simulink model "Ejercicio2_CustomFuzzyBlock"  (R2025a)
settings: Solver=ode8  StartTime=0.0  StopTime=10.0  FixedStep=0.01  RelTol=1e-3
libraries: fuzblock x1
settings Model: Creator=zokra  LastModifiedBy=440G5

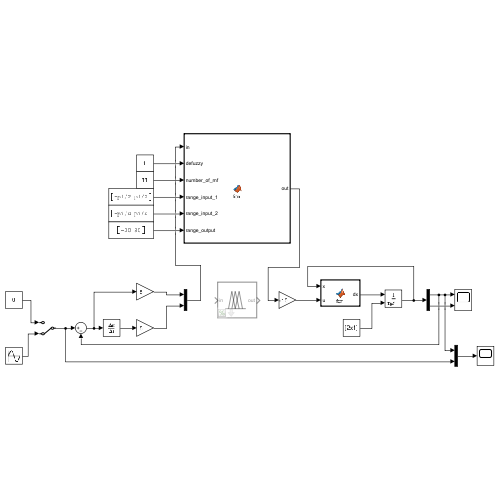
[thumbnail: Simulink's stored preview of the top-level diagram]
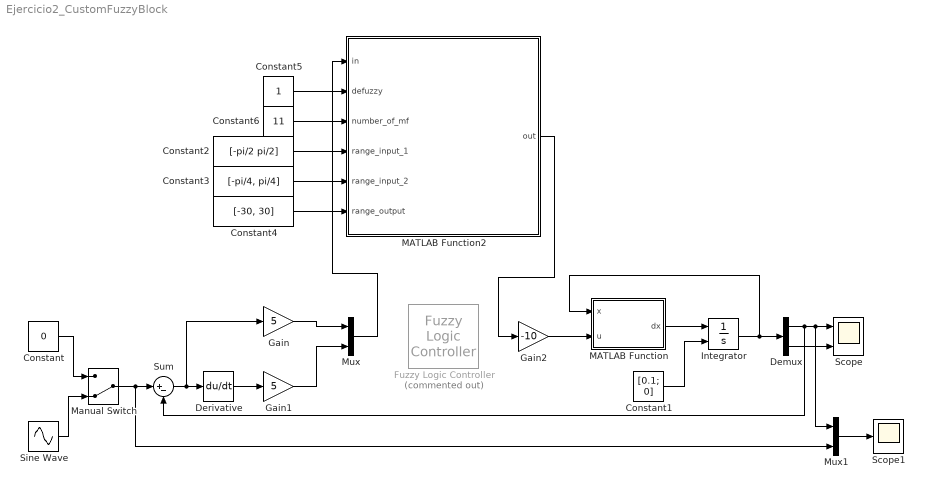
== system Ejercicio2_CustomFuzzyBlock ==
  Constant : Constant  Value=0
  Constant1 : Constant  Value=[0.1; 0]
  Constant2 : Constant  Value=[-pi/2 pi/2]
  Constant3 : Constant  Value=[-pi/4, pi/4]
  Constant4 : Constant  Value=[-30, 30]
  Constant5 : Constant
  Constant6 : Constant  Value=11
  Demux : Demux  Outputs=2
  Derivative : Derivative
  Fuzzy Logic Controller : fuzblock/Fuzzy Logic  Controller  Commented=on  FIS='25_rules_4.fis'  OutputSampleNumber=101  DataType=double  UseLookupTable=off  NumBreakpoints=10  FuzzifiedInputs=off  RuleFiringStrengths=off  RuleOutputs=off  AggregatedOutputs=off  SimulateUsing=Interpreted execution  OutOfRangeInputValueMessage=warning  NoRuleFiredMessage=warning  EmptyOutputFuzzySetMessage=warning
  Gain : Gain  Gain=5
  Gain1 : Gain  Gain=5
  Gain2 : Gain  Gain=-10
  Integrator : Integrator  InitialConditionSource=external
  MATLAB Function : MATLAB Function  TreatAsAtomicUnit=on
  MATLAB Function2 : MATLAB Function  TreatAsAtomicUnit=on
  Manual Switch : ManualSwitch  CurrentSetting=0
  Mux : Mux  Inputs=2
  Mux1 : Mux  Inputs=2
  Scope : Scope  NumInputPorts=2
      settings: ActiveDisplayYMinimum=-1.3075459669239078  ActiveDisplayYMaximum=1.2977307322664664
  Scope1 : Scope
      settings: ActiveDisplayYMinimum=-4.8685764943660805  ActiveDisplayYMaximum=9.3021625081322767
  Sine Wave : Sin  Amplitude=0.25  Frequency=4  SampleTime=0
  Sum : Sum  Inputs=|+-
  wires:
  Derivative/1 -> Gain1/1
  Gain/1 -> Mux/1
  Gain1/1 -> Mux/2
  Integrator/1 -> Demux/1, MATLAB Function/1(x)
  Constant1/1 -> Integrator/2
  Manual Switch/1 -> Mux1/2, Sum/1
  Sum/1 -> Gain/1, Derivative/1
  Mux1/1 -> Scope1/1
  Demux/1 -> Scope/1, Mux1/1, Sum/2
  Demux/2 -> Scope/2
  Sine Wave/1 -> Manual Switch/2
  Constant/1 -> Manual Switch/1
  MATLAB Function/1(dx) -> Integrator/1
  Gain2/1 -> MATLAB Function/2(u)
  Constant4/1 -> MATLAB Function2/6(range_output)
  Constant3/1 -> MATLAB Function2/5(range_input_2)
  Constant2/1 -> MATLAB Function2/4(range_input_1)
  Constant5/1 -> MATLAB Function2/2(defuzzy)
  Mux/1 -> MATLAB Function2/1(in)
  MATLAB Function2/1(out) -> Gain2/1
  Constant6/1 -> MATLAB Function2/3(number_of_mf)

== matlab function Ejercicio2_CustomFuzzyBlock/MATLAB Function ==
  data: x input; u input; dx output
function dx  = fcn(x, u)
g = 9.81;  
l = 1;     
m = 1;     
b = 0.5;   

x1 = x(1);  
x2 = x(2);

dx1 = x2;
dx2 = (g/l)*sin(x1) - (b/(m*l^2))*x2 + u/(m*l^2);

dx = [dx1; dx2];

y = x1;

== matlab function Ejercicio2_CustomFuzzyBlock/MATLAB Function2 ==
  data: in input; out output; defuzzy input; number_of_mf input; range_input_1 input; range_input_2 input; range_output input
function out = fcn(in, defuzzy, number_of_mf, range_input_1, range_input_2, range_output)
% in: [error, d_error]
% defuzzy: 0 = COG, 1 = CA
% range_input_1/2: [min, max]
% range_output: [min, max]

% === 1. Preparar divisiones ===
div1 = linspace(range_input_1(1), range_input_1(2), number_of_mf); % error
div2 = linspace(range_input_2(1), range_input_2(2), number_of_mf); % d_error
div_out = linspace(range_output(1), range_output(2), number_of_mf); % salida

% === 2. Calcular membresías de entrada ===
mu_e = compute_memberships(in(1), div1);
mu_de = compute_memberships(in(2), div2);

% === 3. Definir FAM ===
FAM = zeros(number_of_mf, number_of_mf);
middle_val = (number_of_mf + 1) / 2;
middle_ij = middle_val*2;
for i = 1:number_of_mf
    for j = 1:number_of_mf
        FAM(i,j) = middle_val + middle_ij - (i + j);
        if FAM(i,j) > number_of_mf 
            FAM(i,j) = number_of_mf;
        end
        if FAM(i,j) < 1
            FAM(i,j) = 1;
        end
    end
end

% === 4. Activaciones de reglas ===
rule_heights = zeros(number_of_mf,number_of_mf);
for i = 1:number_of_mf
    for j = 1:number_of_mf
        out_idx = FAM(i,j);
        h = min(mu_e(i), mu_de(j));
        rule_heights(i,j) = h;
    end
end

% Max activación por salida
mu_out = zeros(1,number_of_mf);
for k = 1:number_of_mf
    mu_out(k) = max(rule_heights(FAM==k));
end

% === 5. Defuzzificación ===
if defuzzy == 0
    % COG
    num = 0; den = 0;
    step = div_out(2)-div_out(1);
    base = 2*step; % base total de cada triángulo
    for k = 1:number_of_mf
        h = mu_out(k);
        if h > 0
            % Base efectiva (triángulo truncado horizontalmente)
            top_base = (1-h)*base;
            A = h*(base+top_base)/2; % área del trapecio
            num = num + A*div_out(k);
            den = den + A;
        end
    end
    if den == 0
        out = div_out(3); % centro
    else
        out = num/den;
    end
else
    % CA (Weighted Average by heights)
    num = sum(mu_out .* div_out);
    den = sum(mu_out);
    if den == 0
        out = div_out(3);
    else
        out = num/den;
    end
end
end

% === Membresías ===
function mu = compute_memberships(x, div)
% Devuelve vector de 5 membresías triangulares
n = length(div);
mu = zeros(1,n);

if x <= div(1)
    mu(1) = 1; return
elseif x >= div(end)
    mu(end) = 1; return
end

for i = 1:n-1
    x1 = div(i); x2 = div(i+1);
    if x >= x1 && x <= x2
        mu(i) = (x2 - x)/(x2 - x1);
        mu(i+1) = (x - x1)/(x2 - x1);
        return
    end
end
end
